simulink model "second_part"  (R2020b)
settings: Solver=VariableStepAuto  StartTime=0.0  StopTime=50  RelTol=1e-3
libraries: simulink x2
settings Model: Creator=ilya-  LastModifiedBy=Le tueur

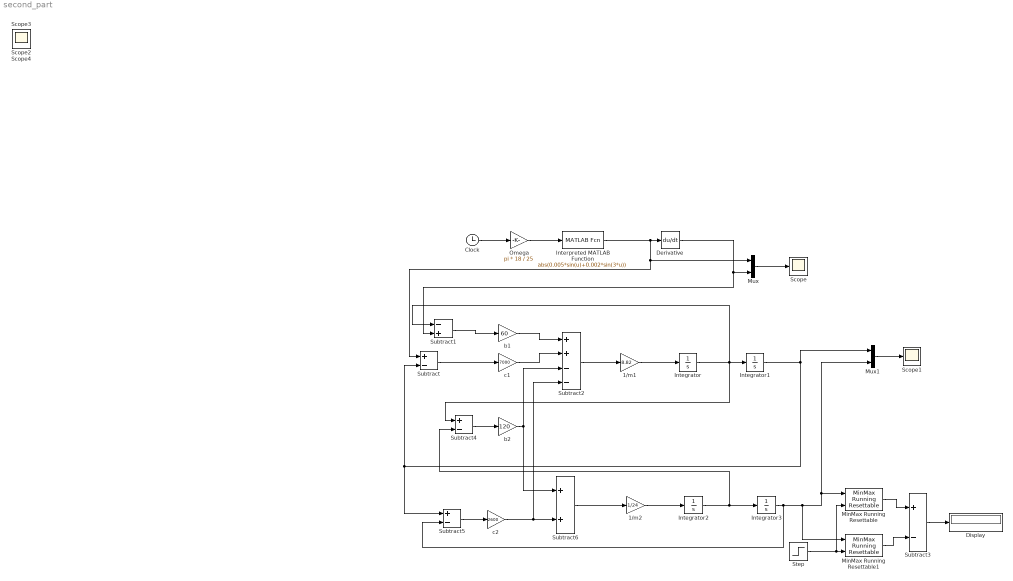
== system second_part ==
  1/m1 : Gain  Gain=8.82
  1/m2 : Gain  Gain=1/24
  Clock : Clock
  Derivative : Derivative
  Display : Display
  Integrator{,1..3} (4 alike) : Integrator
  Interpreted MATLAB Function : MATLABFcn  MATLABFcn=abs(0.005*sin(u)+0.002*sin(3*u))  OutputSignalType=real
  MinMax Running Resettable : simulink/Math Operations/MinMax Running Resettable  Function=max  vinit=0.0
  MinMax Running Resettable1 : simulink/Math Operations/MinMax Running Resettable  Function=min  vinit=10
  Mux : Mux  Inputs=2
  Mux1 : Mux  Inputs=2
  Omega : Gain  Gain=pi * 18 / 25
  Scope{,1..4} (5 alike) : Scope
  Step : Step  Time=20  Before=1  After=0  SampleTime=10
  Subtract{,3..5} (4 alike) : Sum  Inputs=+-
  Subtract1 : Sum  Inputs=-+
  Subtract2 : Sum  Inputs=++--
  Subtract6 : Sum
  b1 : Gain  Gain=60
  b2 : Gain  Gain=120
  c1 : Gain  Gain=7000
  c2 : Gain  Gain=2600
  wires:
  Interpreted MATLAB Function/1 -> Mux/1, Subtract/1, Derivative/1
  Omega/1 -> Interpreted MATLAB Function/1
  Integrator2/1 -> Subtract4/2, Integrator3/1
  b1/1 -> Subtract2/1
  Subtract6/1 -> 1/m2/1
  Integrator3/1 -> Subtract5/2, Mux1/2, MinMax Running Resettable/1, MinMax Running Resettable1/1
  Subtract5/1 -> c2/1
  c1/1 -> Subtract2/2
  Derivative/1 -> Mux/2, Subtract1/2
  1/m2/1 -> Integrator2/1
  Mux1/1 -> Scope1/1
  Clock/1 -> Omega/1
  b2/1 -> Subtract6/1, Subtract2/3
  Subtract1/1 -> b1/1
  Subtract4/1 -> b2/1
  1/m1/1 -> Integrator/1
  Subtract2/1 -> 1/m1/1
  Integrator1/1 -> Mux1/1, Subtract/2, Subtract5/1
  Subtract/1 -> c1/1
  Integrator/1 -> Subtract4/1, Integrator1/1, Subtract1/1
  Mux/1 -> Scope/1
  c2/1 -> Subtract2/4, Subtract6/2
  Step/1 -> MinMax Running Resettable/2, MinMax Running Resettable1/2
  MinMax Running Resettable1/1 -> Subtract3/2
  MinMax Running Resettable/1 -> Subtract3/1
  Subtract3/1 -> Display/1
